simulink model "regelstrecke_simulink"  (R2025b)
settings: Solver=VariableStepAuto  StartTime=0.0  StopTime=10.0  RelTol=1e-3
values from neighbouring files (symbols this model uses):
  final_value = 10    [a1_params.m]    (also in params.m)
  init_value = 0    [a1_params.m]    (also in params.m)
  J = 0.4e9    (= 400000000)    [a1_params.m]    (also in params.m = 0.0004)
  K = 30e-3    (= 0.03)    [a1_params.m]    (also in params.m)
  L = 120e-6    (= 0.00012)    [a1_params.m]    (also in params.m)
  R = 6    [a1_params.m]    (also in params.m)
  sample_time = 0    [a1_params.m]    (also in params.m)
  step_time = 1    [a1_params.m]    (also in params.m = 0)
settings Model: Creator=rishabh  LastModifiedBy=rishabh

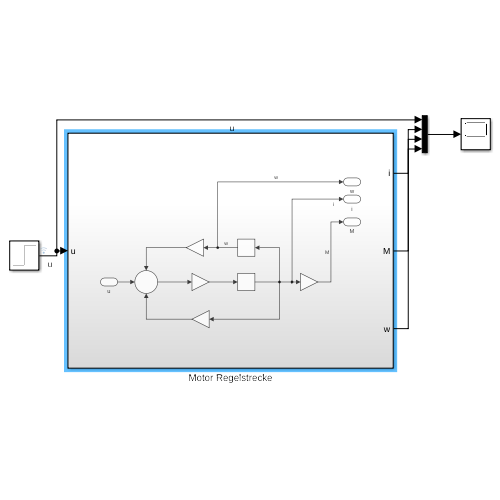
[thumbnail: Simulink's stored preview of the top-level diagram]
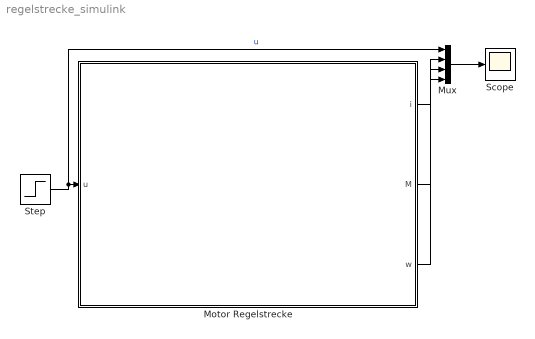
== system regelstrecke_simulink ==
  Motor Regelstrecke : Subsystem
  Mux : Mux
  Scope : Scope
      settings: ActiveDisplayYMinimum=-1.8334341473911169  ActiveDisplayYMaximum=16.500907326520057
  Step : Step  Time=step_time  Before=init_value  After=final_value  SampleTime=sample_time
  wires:
  Step/1 -> Motor Regelstrecke/1(u), Mux/1  "u"
  Mux/1 -> Scope/1
  Motor Regelstrecke/1(i) -> Mux/2
  Motor Regelstrecke/2(M) -> Mux/3
  Motor Regelstrecke/3(w) -> Mux/4

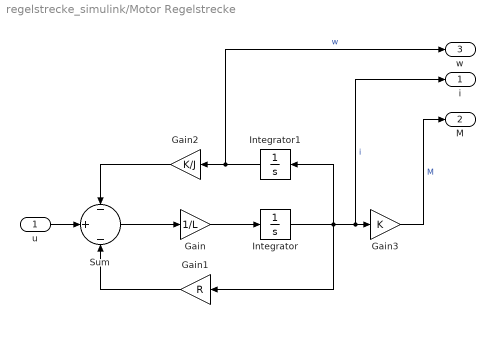
== system regelstrecke_simulink/Motor Regelstrecke ==
  u : Inport
  Gain : Gain  Gain=1/L
  Gain1 : Gain  Gain=R
  Gain2 : Gain  Gain=K/J
  Gain3 : Gain  Gain=K
  Integrator : Integrator
  Integrator1 : Integrator
  Sum : Sum  Inputs=-|+|-
  i : Outport
  M : Outport  Port=2
  w : Outport  Port=3
  wires:
  Sum/1 -> Gain/1
  Gain1/1 -> Sum/3
  Integrator1/1 -> w/1, Gain2/1  "w"
  Integrator/1 -> Gain1/1, Integrator1/1, i/1, Gain3/1  "i"
  Gain2/1 -> Sum/1
  Gain/1 -> Integrator/1
  u/1 -> Sum/2
  Gain3/1 -> M/1  "M"
